simulink model "exp1_water_level"  (R2023a)
settings: Solver=VariableStepAuto  StartTime=0.0  StopTime=20  RelTol=1e-3
model workspace (MAT data in the model file):
  A = [1 1 2 2]
  R = [1 2 1 2]
settings Model: Creator=Nipun_Work  LastModifiedBy=nipun

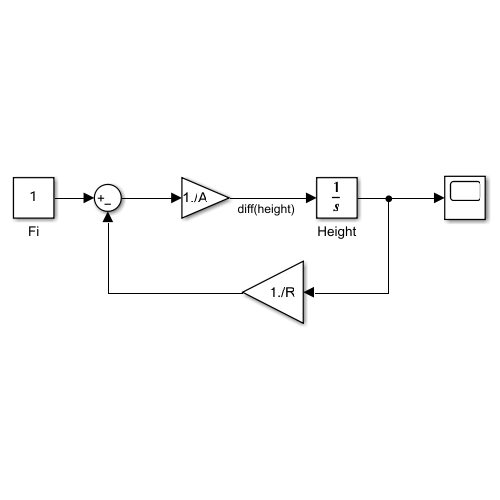
[thumbnail: Simulink's stored preview of the top-level diagram]
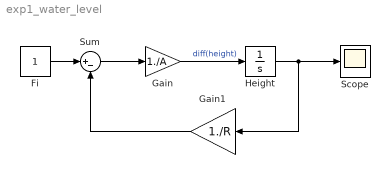
== system exp1_water_level ==
  Fi : Constant
  Gain : Gain  Gain=1./A
  Gain1 : Gain  Gain=1./R
  Height : Integrator
  Scope : Scope
  Sum : Sum  Inputs=|+-
  wires:
  Height/1 -> Gain1/1, Scope/1
  Gain1/1 -> Sum/2
  Gain/1 -> Height/1  "diff(height)"
  Sum/1 -> Gain/1
  Fi/1 -> Sum/1
